simulink model "Viento_coordenadas"  (R2020a)
settings: Solver=VariableStepAuto  StartTime=0.0  StopTime=20  RelTol=1e-3
values from neighbouring files (symbols this model uses):
  Areavector = [0.293;0.022;0.022]    [Iteradorcompleto.m]    (also in Parametros_iniciales.m)
  body_rate_0 = [0;0;0]    [Iteradorcompleto.m]    (also in Parametros_iniciales.m)
  cd = 0.2    [Iteradorcompleto.m]    (also in Parametros_iniciales.m)
  Euler_0 = [0;0;0]    [Iteradorcompleto.m]    (also in Parametros_iniciales.m)
  g = [0;0;-3.66]    [Iteradorcompleto.m]    (also in Parametros_iniciales.m)
  I = [[0.01739,0,0];[0,0.01739,0];[0,0,0.0225]]    [Iteradorcompleto.m]    (also in Parametros_iniciales.m)
  m = T_V1toI*T_V2toV1*T_BtoV2    [Creacion_animacion.m]    (also in Iteradorcompleto.m = 2; Parametros_iniciales.m = 2)
  rho = 0.0195    [Iteradorcompleto.m]    (also in Parametros_iniciales.m)
  ts = 0.01    [Iteradorcompleto.m]    (also in Parametros_iniciales.m)
  vwind = real(-C*(log(1-probabilidad))^(1/K))    [DistribucionWeibul.m]    (also in Iteradorcompleto.m)
  XYZ_0 = [0;0;0]    [Iteradorcompleto.m]    (also in Parametros_iniciales.m = [0;0;5])
libraries: simulink x51, vrlib x2, aerolibutil x1
(part 4 of 4)

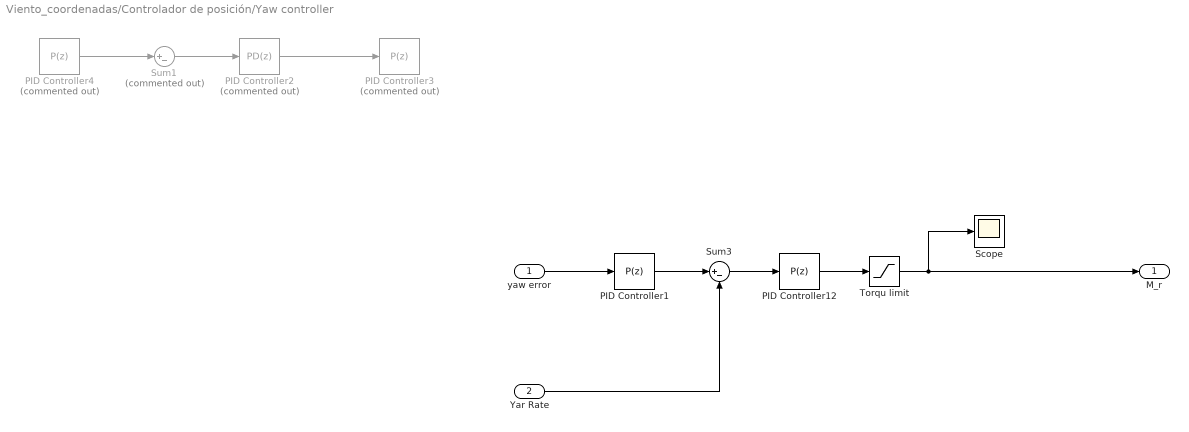
== system Viento_coordenadas/Controlador de posición/Yaw controller  ==
  yaw error : Inport
  Yar Rate : Inport  Port=2
  PID Controller1 : simulink/Continuous/PID Controller  Controller=P  Form=Parallel  TimeDomain=Discrete-time  UseExternalTs=off  SampleTime=ts  IntegratorMethod=Forward Euler  FilterMethod=Forward Euler  ControllerParametersSource=internal  P=4  I=1  D=0  UseFilter=on  N=100  TunerSelectOption=Transfer Function Based (PID Tuner App)  InitialConditionSource=internal  InitialConditionForIntegrator=0  InitialConditionForFilter=0  DifferentiatorICPrevScaledInput=0  ExternalReset=none  TrackingMode=off  Kt=1  LimitOutput=off  UpperSaturationLimit=inf  LowerSaturationLimit=-inf  LinearizeAsGain=on  AntiWindupMode=none  Kb=1  POutMin=[]  POutMax=[]  IOutMin=[]  IOutMax=[]  DOutMin=[]  DOutMax=[]  NOutMin=[]  NOutMax=[]  SumOutMin=[]  SumOutMax=[]  SaturationOutMin=[]  SaturationOutMax=[]  PParamMin=[]  PParamMax=[]  IParamMin=[]  IParamMax=[]  DParamMin=[]  DParamMax=[]  NParamMin=[]  NParamMax=[]  KbParamMin=[]  KbParamMax=[]  KtParamMin=[]  KtParamMax=[]  KbOutMin=[]  KbOutMax=[]  KtOutMin=[]  KtOutMax=[]  IntegratorOutMin=[]  IntegratorOutMax=[]  FilterOutMin=[]  FilterOutMax=[]  SumI1OutMin=[]  SumI1OutMax=[]  SumI2OutMin=[]  SumI2OutMax=[]  SumI3OutMin=[]  SumI3OutMax=[]  SumI4OutMin=[]  SumI4OutMax=[]  SumDOutMin=[]  SumDOutMax=[]  DifferentiatorOutMin=[]  DifferentiatorOutMax=[]  FilterDiffOutCoefMin=[]  FilterDiffOutCoefMax=[]  ReciprocalOutMin=[]  ReciprocalOutMax=[]  SumDenOutMin=[]  SumDenOutMax=[]  SumNumOutMin=[]  SumNumOutMax=[]  DivideOutMin=[]  DivideOutMax=[]  UdiffTsProdOutMin=[]  UdiffTsProdOutMax=[]  NTsProdOutMin=[]  NTsProdOutMax=[]  UintegralTsProdOutMin=[]  UintegralTsProdOutMax=[]  UngainTsProdOutMin=[]  UngainTsProdOutMax=[]  IntegratorContinuousStateAttributes=''  IntegratorStateMustResolveToSignalObject=off  IntegratorRTWStateStorageClass=Auto  FilterContinuousStateAttributes=''  FilterStateMustResolveToSignalObject=off  FilterRTWStateStorageClass=Auto  ParallelPVariant=InternalParameters  IdealPVariant=Disabled  IVariant=Disabled  DVariant=Disabled  IntegratorVariant=Disabled  SatVariant=Disabled  AWVariant=Disabled  PCopyVariant=Disabled  TRVariant=Disabled  FdbkBlocksVariant=Forward  IdealPFdbkVariant=Disabled  SatFdbkVariant=Disabled  DerivativeFilterVariant=Disabled  NVariant=Disabled  NCopyVariant=Disabled_SignalSpec  FilterICVariant=Disabled  IntegratorICVariant=Disabled  ExternalResetVariant=Disabled  TRSumVariant=Passthrough  SumFdbkVariant=Disabled  SumVariant=Passthrough_P  TsampFilterVariant=InternalTs  TsampNgainVariant=Passthrough  TsampIntegralVariant=Disabled_SignalSpec
  PID Controller12 : simulink/Continuous/PID Controller  Controller=P  Form=Parallel  TimeDomain=Discrete-time  UseExternalTs=off  SampleTime=ts  IntegratorMethod=Forward Euler  FilterMethod=Forward Euler  ControllerParametersSource=internal  P=1.5  I=0.0156974923564251  D=-0.0168622468908016  UseFilter=on  N=1.70578345077793  TunerSelectOption=Transfer Function Based (PID Tuner App)  InitialConditionSource=internal  InitialConditionForIntegrator=0  InitialConditionForFilter=0  DifferentiatorICPrevScaledInput=0  ExternalReset=none  TrackingMode=off  Kt=1  LimitOutput=off  UpperSaturationLimit=inf  LowerSaturationLimit=-inf  LinearizeAsGain=on  AntiWindupMode=none  Kb=1  POutMin=[]  POutMax=[]  IOutMin=[]  IOutMax=[]  DOutMin=[]  DOutMax=[]  NOutMin=[]  NOutMax=[]  SumOutMin=[]  SumOutMax=[]  SaturationOutMin=[]  SaturationOutMax=[]  PParamMin=[]  PParamMax=[]  IParamMin=[]  IParamMax=[]  DParamMin=[]  DParamMax=[]  NParamMin=[]  NParamMax=[]  KbParamMin=[]  KbParamMax=[]  KtParamMin=[]  KtParamMax=[]  KbOutMin=[]  KbOutMax=[]  KtOutMin=[]  KtOutMax=[]  IntegratorOutMin=[]  IntegratorOutMax=[]  FilterOutMin=[]  FilterOutMax=[]  SumI1OutMin=[]  SumI1OutMax=[]  SumI2OutMin=[]  SumI2OutMax=[]  SumI3OutMin=[]  SumI3OutMax=[]  SumI4OutMin=[]  SumI4OutMax=[]  SumDOutMin=[]  SumDOutMax=[]  DifferentiatorOutMin=[]  DifferentiatorOutMax=[]  FilterDiffOutCoefMin=[]  FilterDiffOutCoefMax=[]  ReciprocalOutMin=[]  ReciprocalOutMax=[]  SumDenOutMin=[]  SumDenOutMax=[]  SumNumOutMin=[]  SumNumOutMax=[]  DivideOutMin=[]  DivideOutMax=[]  UdiffTsProdOutMin=[]  UdiffTsProdOutMax=[]  NTsProdOutMin=[]  NTsProdOutMax=[]  UintegralTsProdOutMin=[]  UintegralTsProdOutMax=[]  UngainTsProdOutMin=[]  UngainTsProdOutMax=[]  IntegratorContinuousStateAttributes=''  IntegratorStateMustResolveToSignalObject=off  IntegratorRTWStateStorageClass=Auto  FilterContinuousStateAttributes=''  FilterStateMustResolveToSignalObject=off  FilterRTWStateStorageClass=Auto  ParallelPVariant=InternalParameters  IdealPVariant=Disabled  IVariant=Disabled  DVariant=Disabled  IntegratorVariant=Disabled  SatVariant=Disabled  AWVariant=Disabled  PCopyVariant=Disabled  TRVariant=Disabled  FdbkBlocksVariant=Forward  IdealPFdbkVariant=Disabled  SatFdbkVariant=Disabled  DerivativeFilterVariant=Disabled  NVariant=Disabled  NCopyVariant=Disabled_SignalSpec  FilterICVariant=Disabled  IntegratorICVariant=Disabled  ExternalResetVariant=Disabled  TRSumVariant=Passthrough  SumFdbkVariant=Disabled  SumVariant=Passthrough_P  TsampFilterVariant=InternalTs  TsampNgainVariant=Passthrough  TsampIntegralVariant=Disabled_SignalSpec
  PID Controller2 : simulink/Continuous/PID Controller  Commented=on  Controller=PD  Form=Parallel  TimeDomain=Discrete-time  UseExternalTs=off  SampleTime=ts  IntegratorMethod=Forward Euler  FilterMethod=Forward Euler  ControllerParametersSource=internal  P=06  I=1  D=0.4  UseFilter=on  N=10  TunerSelectOption=Transfer Function Based (PID Tuner App)  InitialConditionSource=internal  InitialConditionForIntegrator=0  InitialConditionForFilter=0  DifferentiatorICPrevScaledInput=0  ExternalReset=none  TrackingMode=off  Kt=1  LimitOutput=off  UpperSaturationLimit=inf  LowerSaturationLimit=-inf  LinearizeAsGain=on  AntiWindupMode=none  Kb=1  POutMin=[]  POutMax=[]  IOutMin=[]  IOutMax=[]  DOutMin=[]  DOutMax=[]  NOutMin=[]  NOutMax=[]  SumOutMin=[]  SumOutMax=[]  SaturationOutMin=[]  SaturationOutMax=[]  PParamMin=[]  PParamMax=[]  IParamMin=[]  IParamMax=[]  DParamMin=[]  DParamMax=[]  NParamMin=[]  NParamMax=[]  KbParamMin=[]  KbParamMax=[]  KtParamMin=[]  KtParamMax=[]  KbOutMin=[]  KbOutMax=[]  KtOutMin=[]  KtOutMax=[]  IntegratorOutMin=[]  IntegratorOutMax=[]  FilterOutMin=[]  FilterOutMax=[]  SumI1OutMin=[]  SumI1OutMax=[]  SumI2OutMin=[]  SumI2OutMax=[]  SumI3OutMin=[]  SumI3OutMax=[]  SumI4OutMin=[]  SumI4OutMax=[]  SumDOutMin=[]  SumDOutMax=[]  DifferentiatorOutMin=[]  DifferentiatorOutMax=[]  FilterDiffOutCoefMin=[]  FilterDiffOutCoefMax=[]  ReciprocalOutMin=[]  ReciprocalOutMax=[]  SumDenOutMin=[]  SumDenOutMax=[]  SumNumOutMin=[]  SumNumOutMax=[]  DivideOutMin=[]  DivideOutMax=[]  UdiffTsProdOutMin=[]  UdiffTsProdOutMax=[]  NTsProdOutMin=[]  NTsProdOutMax=[]  UintegralTsProdOutMin=[]  UintegralTsProdOutMax=[]  UngainTsProdOutMin=[]  UngainTsProdOutMax=[]  IntegratorContinuousStateAttributes=''  IntegratorStateMustResolveToSignalObject=off  IntegratorRTWStateStorageClass=Auto  FilterContinuousStateAttributes=''  FilterStateMustResolveToSignalObject=off  FilterRTWStateStorageClass=Auto  ParallelPVariant=InternalParameters  IdealPVariant=Disabled  IVariant=Disabled  DVariant=InternalParameters  IntegratorVariant=Disabled  SatVariant=Disabled  AWVariant=Disabled  PCopyVariant=Disabled  TRVariant=Disabled  FdbkBlocksVariant=Forward  IdealPFdbkVariant=Disabled  SatFdbkVariant=Disabled  DerivativeFilterVariant=ForwardEulerFilter  NVariant=InternalParameters  NCopyVariant=Disabled  FilterICVariant=InternalICsFilter  IntegratorICVariant=Disabled  ExternalResetVariant=Disabled  TRSumVariant=Passthrough  SumFdbkVariant=Disabled  SumVariant=Sum_PD  TsampFilterVariant=InternalTs  TsampNgainVariant=Passthrough  TsampIntegralVariant=Disabled_SignalSpec
  PID Controller3 : simulink/Continuous/PID Controller  Commented=on  Controller=P  Form=Parallel  TimeDomain=Discrete-time  UseExternalTs=off  SampleTime=ts  IntegratorMethod=Forward Euler  FilterMethod=Forward Euler  ControllerParametersSource=internal  P=0.7  I=1  D=0  UseFilter=on  N=100  TunerSelectOption=Transfer Function Based (PID Tuner App)  InitialConditionSource=internal  InitialConditionForIntegrator=0  InitialConditionForFilter=0  DifferentiatorICPrevScaledInput=0  ExternalReset=none  TrackingMode=off  Kt=1  LimitOutput=off  UpperSaturationLimit=inf  LowerSaturationLimit=-inf  LinearizeAsGain=on  AntiWindupMode=none  Kb=1  POutMin=[]  POutMax=[]  IOutMin=[]  IOutMax=[]  DOutMin=[]  DOutMax=[]  NOutMin=[]  NOutMax=[]  SumOutMin=[]  SumOutMax=[]  SaturationOutMin=[]  SaturationOutMax=[]  PParamMin=[]  PParamMax=[]  IParamMin=[]  IParamMax=[]  DParamMin=[]  DParamMax=[]  NParamMin=[]  NParamMax=[]  KbParamMin=[]  KbParamMax=[]  KtParamMin=[]  KtParamMax=[]  KbOutMin=[]  KbOutMax=[]  KtOutMin=[]  KtOutMax=[]  IntegratorOutMin=[]  IntegratorOutMax=[]  FilterOutMin=[]  FilterOutMax=[]  SumI1OutMin=[]  SumI1OutMax=[]  SumI2OutMin=[]  SumI2OutMax=[]  SumI3OutMin=[]  SumI3OutMax=[]  SumI4OutMin=[]  SumI4OutMax=[]  SumDOutMin=[]  SumDOutMax=[]  DifferentiatorOutMin=[]  DifferentiatorOutMax=[]  FilterDiffOutCoefMin=[]  FilterDiffOutCoefMax=[]  ReciprocalOutMin=[]  ReciprocalOutMax=[]  SumDenOutMin=[]  SumDenOutMax=[]  SumNumOutMin=[]  SumNumOutMax=[]  DivideOutMin=[]  DivideOutMax=[]  UdiffTsProdOutMin=[]  UdiffTsProdOutMax=[]  NTsProdOutMin=[]  NTsProdOutMax=[]  UintegralTsProdOutMin=[]  UintegralTsProdOutMax=[]  UngainTsProdOutMin=[]  UngainTsProdOutMax=[]  IntegratorContinuousStateAttributes=''  IntegratorStateMustResolveToSignalObject=off  IntegratorRTWStateStorageClass=Auto  FilterContinuousStateAttributes=''  FilterStateMustResolveToSignalObject=off  FilterRTWStateStorageClass=Auto  ParallelPVariant=InternalParameters  IdealPVariant=Disabled  IVariant=Disabled  DVariant=Disabled  IntegratorVariant=Disabled  SatVariant=Disabled  AWVariant=Disabled  PCopyVariant=Disabled  TRVariant=Disabled  FdbkBlocksVariant=Forward  IdealPFdbkVariant=Disabled  SatFdbkVariant=Disabled  DerivativeFilterVariant=Disabled  NVariant=Disabled  NCopyVariant=Disabled_SignalSpec  FilterICVariant=Disabled  IntegratorICVariant=Disabled  ExternalResetVariant=Disabled  TRSumVariant=Passthrough  SumFdbkVariant=Disabled  SumVariant=Passthrough_P  TsampFilterVariant=InternalTs  TsampNgainVariant=Passthrough  TsampIntegralVariant=Disabled_SignalSpec
  PID Controller4 : simulink/Continuous/PID Controller  Commented=on  Controller=P  Form=Parallel  TimeDomain=Discrete-time  UseExternalTs=off  SampleTime=ts  IntegratorMethod=Forward Euler  FilterMethod=Forward Euler  ControllerParametersSource=internal  P=6  I=1  D=0  UseFilter=on  N=100  TunerSelectOption=Transfer Function Based (PID Tuner App)  InitialConditionSource=internal  InitialConditionForIntegrator=0  InitialConditionForFilter=0  DifferentiatorICPrevScaledInput=0  ExternalReset=none  TrackingMode=off  Kt=1  LimitOutput=off  UpperSaturationLimit=inf  LowerSaturationLimit=-inf  LinearizeAsGain=on  AntiWindupMode=none  Kb=1  POutMin=[]  POutMax=[]  IOutMin=[]  IOutMax=[]  DOutMin=[]  DOutMax=[]  NOutMin=[]  NOutMax=[]  SumOutMin=[]  SumOutMax=[]  SaturationOutMin=[]  SaturationOutMax=[]  PParamMin=[]  PParamMax=[]  IParamMin=[]  IParamMax=[]  DParamMin=[]  DParamMax=[]  NParamMin=[]  NParamMax=[]  KbParamMin=[]  KbParamMax=[]  KtParamMin=[]  KtParamMax=[]  KbOutMin=[]  KbOutMax=[]  KtOutMin=[]  KtOutMax=[]  IntegratorOutMin=[]  IntegratorOutMax=[]  FilterOutMin=[]  FilterOutMax=[]  SumI1OutMin=[]  SumI1OutMax=[]  SumI2OutMin=[]  SumI2OutMax=[]  SumI3OutMin=[]  SumI3OutMax=[]  SumI4OutMin=[]  SumI4OutMax=[]  SumDOutMin=[]  SumDOutMax=[]  DifferentiatorOutMin=[]  DifferentiatorOutMax=[]  FilterDiffOutCoefMin=[]  FilterDiffOutCoefMax=[]  ReciprocalOutMin=[]  ReciprocalOutMax=[]  SumDenOutMin=[]  SumDenOutMax=[]  SumNumOutMin=[]  SumNumOutMax=[]  DivideOutMin=[]  DivideOutMax=[]  UdiffTsProdOutMin=[]  UdiffTsProdOutMax=[]  NTsProdOutMin=[]  NTsProdOutMax=[]  UintegralTsProdOutMin=[]  UintegralTsProdOutMax=[]  UngainTsProdOutMin=[]  UngainTsProdOutMax=[]  IntegratorContinuousStateAttributes=''  IntegratorStateMustResolveToSignalObject=off  IntegratorRTWStateStorageClass=Auto  FilterContinuousStateAttributes=''  FilterStateMustResolveToSignalObject=off  FilterRTWStateStorageClass=Auto  ParallelPVariant=InternalParameters  IdealPVariant=Disabled  IVariant=Disabled  DVariant=Disabled  IntegratorVariant=Disabled  SatVariant=Disabled  AWVariant=Disabled  PCopyVariant=Disabled  TRVariant=Disabled  FdbkBlocksVariant=Forward  IdealPFdbkVariant=Disabled  SatFdbkVariant=Disabled  DerivativeFilterVariant=Disabled  NVariant=Disabled  NCopyVariant=Disabled_SignalSpec  FilterICVariant=Disabled  IntegratorICVariant=Disabled  ExternalResetVariant=Disabled  TRSumVariant=Passthrough  SumFdbkVariant=Disabled  SumVariant=Passthrough_P  TsampFilterVariant=InternalTs  TsampNgainVariant=Passthrough  TsampIntegralVariant=Disabled_SignalSpec
  Scope : Scope
  Sum1 : Sum  Commented=on  Inputs=|+-
  Sum3 : Sum  Inputs=|+-
  Torqu limit : Saturate  UpperLimit=1  LowerLimit=-1
  M_r : Outport
  wires:
  PID Controller12/1 -> Torqu limit/1
  Sum3/1 -> PID Controller12/1
  PID Controller1/1 -> Sum3/1
  Torqu limit/1 -> M_r/1, Scope/1
  PID Controller4/1 -> Sum1/1
  Sum1/1 -> PID Controller2/1
  PID Controller2/1 -> PID Controller3/1
  yaw error/1 -> PID Controller1/1
  Yar Rate/1 -> Sum3/2

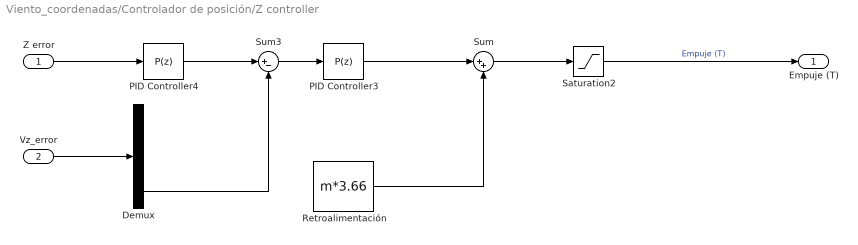
== system Viento_coordenadas/Controlador de posición/Z controller ==
  Z error : Inport
  Vz_error : Inport  Port=2
  Demux : Demux  Outputs=3
  PID Controller3 : simulink/Continuous/PID Controller  Controller=P  Form=Parallel  TimeDomain=Discrete-time  UseExternalTs=off  SampleTime=ts  IntegratorMethod=Forward Euler  FilterMethod=Forward Euler  ControllerParametersSource=internal  P=1.5  I=1  D=0  UseFilter=on  N=100  TunerSelectOption=Transfer Function Based (PID Tuner App)  InitialConditionSource=internal  InitialConditionForIntegrator=0  InitialConditionForFilter=0  DifferentiatorICPrevScaledInput=0  ExternalReset=none  TrackingMode=off  Kt=1  LimitOutput=off  UpperSaturationLimit=inf  LowerSaturationLimit=-inf  LinearizeAsGain=on  AntiWindupMode=none  Kb=1  POutMin=[]  POutMax=[]  IOutMin=[]  IOutMax=[]  DOutMin=[]  DOutMax=[]  NOutMin=[]  NOutMax=[]  SumOutMin=[]  SumOutMax=[]  SaturationOutMin=[]  SaturationOutMax=[]  PParamMin=[]  PParamMax=[]  IParamMin=[]  IParamMax=[]  DParamMin=[]  DParamMax=[]  NParamMin=[]  NParamMax=[]  KbParamMin=[]  KbParamMax=[]  KtParamMin=[]  KtParamMax=[]  KbOutMin=[]  KbOutMax=[]  KtOutMin=[]  KtOutMax=[]  IntegratorOutMin=[]  IntegratorOutMax=[]  FilterOutMin=[]  FilterOutMax=[]  SumI1OutMin=[]  SumI1OutMax=[]  SumI2OutMin=[]  SumI2OutMax=[]  SumI3OutMin=[]  SumI3OutMax=[]  SumI4OutMin=[]  SumI4OutMax=[]  SumDOutMin=[]  SumDOutMax=[]  DifferentiatorOutMin=[]  DifferentiatorOutMax=[]  FilterDiffOutCoefMin=[]  FilterDiffOutCoefMax=[]  ReciprocalOutMin=[]  ReciprocalOutMax=[]  SumDenOutMin=[]  SumDenOutMax=[]  SumNumOutMin=[]  SumNumOutMax=[]  DivideOutMin=[]  DivideOutMax=[]  UdiffTsProdOutMin=[]  UdiffTsProdOutMax=[]  NTsProdOutMin=[]  NTsProdOutMax=[]  UintegralTsProdOutMin=[]  UintegralTsProdOutMax=[]  UngainTsProdOutMin=[]  UngainTsProdOutMax=[]  IntegratorContinuousStateAttributes=''  IntegratorStateMustResolveToSignalObject=off  IntegratorRTWStateStorageClass=Auto  FilterContinuousStateAttributes=''  FilterStateMustResolveToSignalObject=off  FilterRTWStateStorageClass=Auto  ParallelPVariant=InternalParameters  IdealPVariant=Disabled  IVariant=Disabled  DVariant=Disabled  IntegratorVariant=Disabled  SatVariant=Disabled  AWVariant=Disabled  PCopyVariant=Disabled  TRVariant=Disabled  FdbkBlocksVariant=Forward  IdealPFdbkVariant=Disabled  SatFdbkVariant=Disabled  DerivativeFilterVariant=Disabled  NVariant=Disabled  NCopyVariant=Disabled_SignalSpec  FilterICVariant=Disabled  IntegratorICVariant=Disabled  ExternalResetVariant=Disabled  TRSumVariant=Passthrough  SumFdbkVariant=Disabled  SumVariant=Passthrough_P  TsampFilterVariant=InternalTs  TsampNgainVariant=Passthrough  TsampIntegralVariant=Disabled_SignalSpec
  PID Controller4 : simulink/Continuous/PID Controller  Controller=P  Form=Parallel  TimeDomain=Discrete-time  UseExternalTs=off  SampleTime=ts  IntegratorMethod=Forward Euler  FilterMethod=Forward Euler  ControllerParametersSource=internal  P=0.4  I=1  D=0  UseFilter=on  N=100  TunerSelectOption=Transfer Function Based (PID Tuner App)  InitialConditionSource=internal  InitialConditionForIntegrator=0  InitialConditionForFilter=0  DifferentiatorICPrevScaledInput=0  ExternalReset=none  TrackingMode=off  Kt=1  LimitOutput=off  UpperSaturationLimit=inf  LowerSaturationLimit=-inf  LinearizeAsGain=on  AntiWindupMode=none  Kb=1  POutMin=[]  POutMax=[]  IOutMin=[]  IOutMax=[]  DOutMin=[]  DOutMax=[]  NOutMin=[]  NOutMax=[]  SumOutMin=[]  SumOutMax=[]  SaturationOutMin=[]  SaturationOutMax=[]  PParamMin=[]  PParamMax=[]  IParamMin=[]  IParamMax=[]  DParamMin=[]  DParamMax=[]  NParamMin=[]  NParamMax=[]  KbParamMin=[]  KbParamMax=[]  KtParamMin=[]  KtParamMax=[]  KbOutMin=[]  KbOutMax=[]  KtOutMin=[]  KtOutMax=[]  IntegratorOutMin=[]  IntegratorOutMax=[]  FilterOutMin=[]  FilterOutMax=[]  SumI1OutMin=[]  SumI1OutMax=[]  SumI2OutMin=[]  SumI2OutMax=[]  SumI3OutMin=[]  SumI3OutMax=[]  SumI4OutMin=[]  SumI4OutMax=[]  SumDOutMin=[]  SumDOutMax=[]  DifferentiatorOutMin=[]  DifferentiatorOutMax=[]  FilterDiffOutCoefMin=[]  FilterDiffOutCoefMax=[]  ReciprocalOutMin=[]  ReciprocalOutMax=[]  SumDenOutMin=[]  SumDenOutMax=[]  SumNumOutMin=[]  SumNumOutMax=[]  DivideOutMin=[]  DivideOutMax=[]  UdiffTsProdOutMin=[]  UdiffTsProdOutMax=[]  NTsProdOutMin=[]  NTsProdOutMax=[]  UintegralTsProdOutMin=[]  UintegralTsProdOutMax=[]  UngainTsProdOutMin=[]  UngainTsProdOutMax=[]  IntegratorContinuousStateAttributes=''  IntegratorStateMustResolveToSignalObject=off  IntegratorRTWStateStorageClass=Auto  FilterContinuousStateAttributes=''  FilterStateMustResolveToSignalObject=off  FilterRTWStateStorageClass=Auto  ParallelPVariant=InternalParameters  IdealPVariant=Disabled  IVariant=Disabled  DVariant=Disabled  IntegratorVariant=Disabled  SatVariant=Disabled  AWVariant=Disabled  PCopyVariant=Disabled  TRVariant=Disabled  FdbkBlocksVariant=Forward  IdealPFdbkVariant=Disabled  SatFdbkVariant=Disabled  DerivativeFilterVariant=Disabled  NVariant=Disabled  NCopyVariant=Disabled_SignalSpec  FilterICVariant=Disabled  IntegratorICVariant=Disabled  ExternalResetVariant=Disabled  TRSumVariant=Passthrough  SumFdbkVariant=Disabled  SumVariant=Passthrough_P  TsampFilterVariant=InternalTs  TsampNgainVariant=Passthrough  TsampIntegralVariant=Disabled_SignalSpec
  "Retroalimentación " : Constant  Value=m*3.66
  Saturation2 : Saturate  UpperLimit=11.396  LowerLimit=-11.396
  Sum : Sum  Inputs=|++
  Sum3 : Sum  Inputs=|+-
  Empuje (T) : Outport
  wires:
  PID Controller4/1 -> Sum3/1
  Sum3/1 -> PID Controller3/1
  Demux/3 -> Sum3/2
  Saturation2/1 -> Empuje (T)/1  "Empuje (T)"
  Sum/1 -> Saturation2/1
  "Retroalimentación "/1 -> Sum/2
  Z error/1 -> PID Controller4/1
  Vz_error/1 -> Demux/1
  PID Controller3/1 -> Sum/1

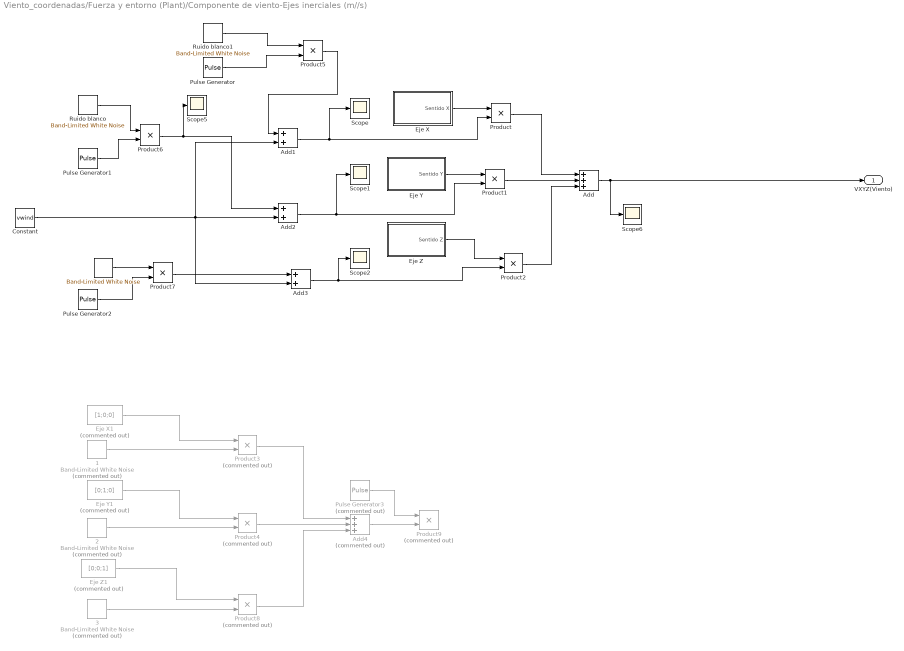
== system Viento_coordenadas/Fuerza y entorno (Plant)/Componente de viento-Ejes inerciales (m//s) ==
  " " : simulink/Sources/Band-Limited White Noise  Cov=[0.05]  Ts=10  seed=[13244]
  " 1" : simulink/Sources/Band-Limited White Noise  Commented=on  Cov=[0.05]  Ts=10  seed=[13244]
  " 2" : simulink/Sources/Band-Limited White Noise  Commented=on  Cov=[0.05]  Ts=10  seed=[13244]
  " 3" : simulink/Sources/Band-Limited White Noise  Commented=on  Cov=[0.05]  Ts=10  seed=[13244]
  Add : Sum  Inputs=+++
  Add1 : Sum
  Add2 : Sum
  Add3 : Sum
  Add4 : Sum  Commented=on  Inputs=+++
  Constant : Constant  Value=vwind
  Eje X : Subsystem
  Eje X1 : Constant  Commented=on  Value=[1;0;0]
  Eje Y : Subsystem
  Eje Y1 : Constant  Commented=on  Value=[0;1;0]
  Eje Z : Subsystem
  Eje Z1 : Constant  Commented=on  Value=[0;0;1]
  Product{,1..2,5..7} (6 alike) : Product
  Product{3..4,8..9} (4 alike) : Product  Commented=on
  Pulse Generator : DiscretePulseGenerator  PulseType=Time based  Amplitude=0.5  Period=5  PulseWidth=20
  Pulse Generator1 : DiscretePulseGenerator  PulseType=Time based  Period=5  PulseWidth=25
  Pulse Generator2 : DiscretePulseGenerator  PulseType=Time based  Amplitude=0.5  Period=5  PulseWidth=17
  Pulse Generator3 : DiscretePulseGenerator  Commented=on  PulseType=Time based  Period=5  PulseWidth=90
  Ruido blanco : simulink/Sources/Band-Limited White Noise  Cov=[0.05]  Ts=7  seed=[23341]
  Ruido blanco1 : simulink/Sources/Band-Limited White Noise  Cov=[0.05]  Ts=5  seed=[23341]
  Scope{,1..2,5..6} (5 alike) : Scope
  VXYZ(Viento) : Outport
  wires:
  Product/1 -> Add/1
  Constant/1 -> Add3/2, Add2/2, Add1/2
  Add1/1 -> Scope/1, Product/2
  Add2/1 -> Scope1/1, Product1/2
  Add3/1 -> Scope2/1, Product2/2
  Ruido blanco1/1 -> Product5/1
  Pulse Generator/1 -> Product5/2
  Product5/1 -> Add1/1
  Ruido blanco/1 -> Product6/1
  Product6/1 -> Scope5/1, Add2/1
  " "/1 -> Product7/1
  Product7/1 -> Add3/1
  Pulse Generator1/1 -> Product6/2
  Pulse Generator2/1 -> Product7/2
  " 1"/1 -> Product3/2
  Eje X1/1 -> Product3/1
  " 2"/1 -> Product4/2
  Eje Y1/1 -> Product4/1
  " 3"/1 -> Product8/2
  Eje Z1/1 -> Product8/1
  Product4/1 -> Add4/2
  Product3/1 -> Add4/1
  Product8/1 -> Add4/3
  Add4/1 -> Product9/2
  Pulse Generator3/1 -> Product9/1
  Add/1 -> Scope6/1, VXYZ(Viento)/1
  Eje X/1(Sentido X) -> Product/1
  Eje Y/1(Sentido Y) -> Product1/1
  Eje Z/1(Sentido Z) -> Product2/1
  Product1/1 -> Add/2
  Product2/1 -> Add/3

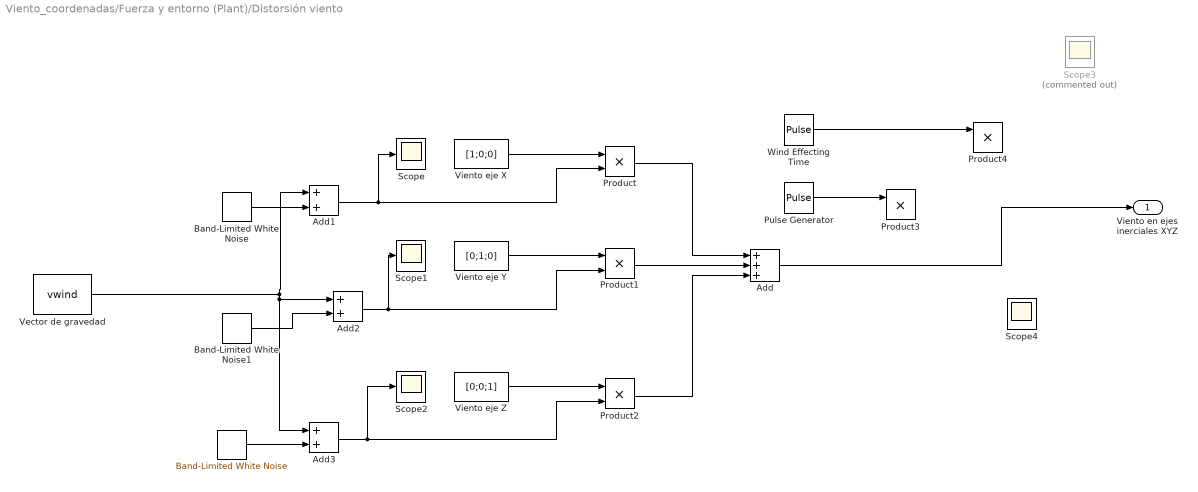
== system Viento_coordenadas/Fuerza y entorno (Plant)/Distorsión viento ==
  " " : simulink/Sources/Band-Limited White Noise  Cov=[0.5]  Ts=5  seed=[13244]
  Add : Sum  Inputs=+++
  Add1 : Sum
  Add2 : Sum
  Add3 : Sum
  Band-Limited White Noise : simulink/Sources/Band-Limited White Noise  Cov=[0.5]  Ts=5  seed=[23341]
  Band-Limited White Noise1 : simulink/Sources/Band-Limited White Noise  Cov=[0.5]  Ts=5  seed=[41323]
  Product{,1..4} (5 alike) : Product
  Pulse Generator : DiscretePulseGenerator  PulseType=Time based  Period=2.5  PulseWidth=40
  Scope{,1..2,4} (4 alike) : Scope
  Scope3 : Scope  Commented=on
  Vector de gravedad : Constant  Value=vwind  SampleTime=-1
  Viento eje X : Constant  Value=[1;0;0]
  Viento eje Y : Constant  Value=[0;1;0]
  Viento eje Z : Constant  Value=[0;0;1]
  Wind Effecting Time : DiscretePulseGenerator  PulseType=Time based  Period=100  PulseWidth=10
  Viento en ejes inerciales XYZ : Outport
  wires:
  Viento eje X/1 -> Product/1
  Viento eje Y/1 -> Product1/1
  Viento eje Z/1 -> Product2/1
  Product1/1 -> Add/2
  Product/1 -> Add/1
  Product2/1 -> Add/3
  Pulse Generator/1 -> Product3/1
  Wind Effecting Time/1 -> Product4/1
  Add/1 -> Viento en ejes inerciales XYZ/1
  Band-Limited White Noise/1 -> Add1/2
  Add1/1 -> Scope/1, Product/2
  Band-Limited White Noise1/1 -> Add2/2
  Add2/1 -> Scope1/1, Product1/2
  " "/1 -> Add3/2
  Add3/1 -> Scope2/1, Product2/2
  Vector de gravedad/1 -> Add3/1, Add2/1, Add1/1

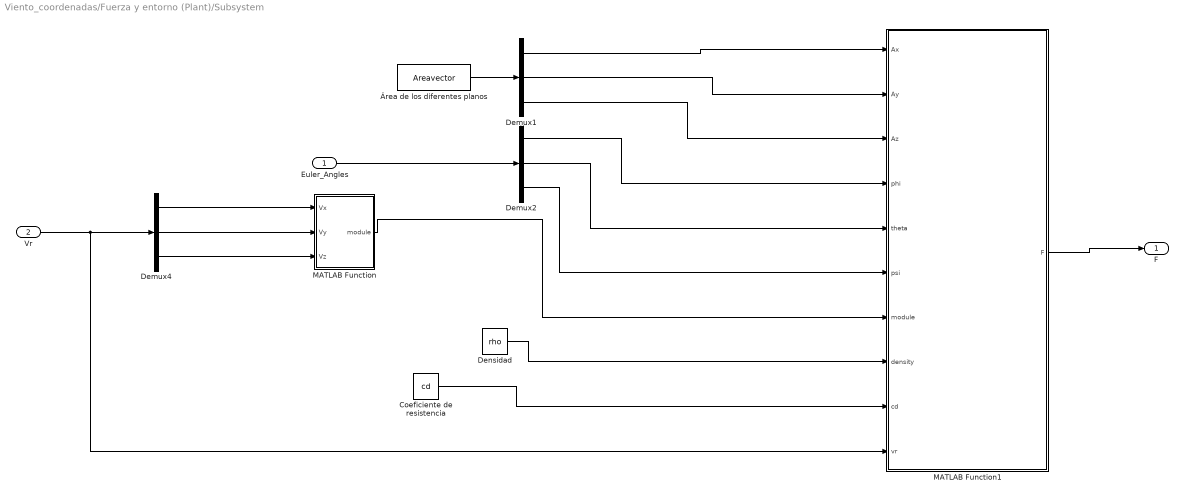
== system Viento_coordenadas/Fuerza y entorno (Plant)/Subsystem ==
  Euler_Angles : Inport
  Vr : Inport  Port=2
  Coeficiente de resistencia : Constant  Value=cd  SampleTime=-1
  Demux1 : Demux  Outputs=3
  Demux2 : Demux  Outputs=3
  Demux4 : Demux  Outputs=3
  Densidad : Constant  Value=rho  SampleTime=-1
  MATLAB Function : MATLAB Function  TreatAsAtomicUnit=on
  MATLAB Function1 : MATLAB Function  TreatAsAtomicUnit=on
  Área de los diferentes planos : Constant  Value=Areavector  SampleTime=-1
  F : Outport
  wires:
  Demux4/3 -> MATLAB Function/3(Vz)
  Demux4/2 -> MATLAB Function/2(Vy)
  Demux2/3 -> MATLAB Function1/6(psi)
  MATLAB Function1/1(F) -> F/1
  Área de los diferentes planos/1 -> Demux1/1
  Demux1/2 -> MATLAB Function1/2(Ay)
  Demux1/3 -> MATLAB Function1/3(Az)
  Euler_Angles/1 -> Demux2/1
  Demux1/1 -> MATLAB Function1/1(Ax)
  Demux2/1 -> MATLAB Function1/4(phi)
  Demux2/2 -> MATLAB Function1/5(theta)
  MATLAB Function/1(module) -> MATLAB Function1/7(module)
  Densidad/1 -> MATLAB Function1/8(density)
  Vr/1 -> Demux4/1, MATLAB Function1/10(vr)
  Demux4/1 -> MATLAB Function/1(Vx)
  Coeficiente de resistencia/1 -> MATLAB Function1/9(cd)

== system Viento_coordenadas/Fuerza y entorno (Plant)/Componente de viento-Ejes inerciales (m//s)/Eje X ==
  Eje X : Constant  Value=[-1;0;0]
  Eje X2 : Constant  Value=[-1;0;0]
  Product : Product
  Pulse Generator : DiscretePulseGenerator  PulseType=Time based  Amplitude=0.5  Period=10  PulseWidth=80
  Ruido blanco2 : simulink/Sources/Band-Limited White Noise  Cov=[0.05]  Ts=6  seed=[23341]
  Switch : Switch  Criteria=u2 > Threshold  Threshold=0.01
  Sentido X : Outport
  wires:
  Ruido blanco2/1 -> Product/1
  Pulse Generator/1 -> Product/2
  Switch/1 -> Sentido X/1
  Eje X/1 -> Switch/1
  Eje X2/1 -> Switch/3
  Product/1 -> Switch/2

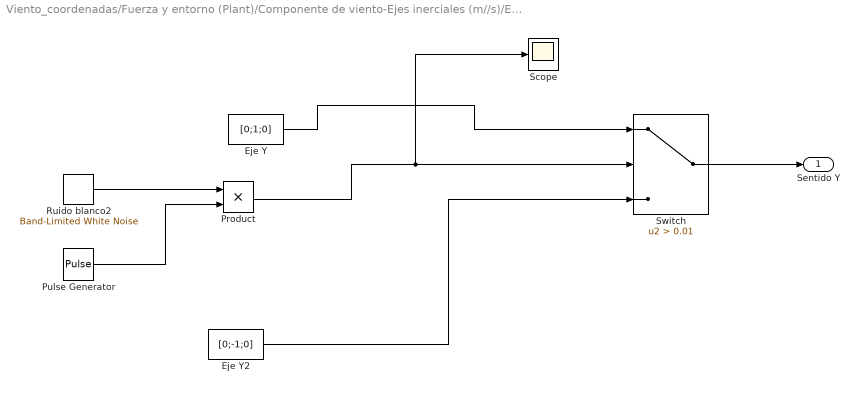
== system Viento_coordenadas/Fuerza y entorno (Plant)/Componente de viento-Ejes inerciales (m//s)/Eje Y ==
  Eje Y : Constant  Value=[0;1;0]
  Eje Y2 : Constant  Value=[0;-1;0]
  Product : Product
  Pulse Generator : DiscretePulseGenerator  PulseType=Time based  Amplitude=0.5  Period=10  PulseWidth=80
  Ruido blanco2 : simulink/Sources/Band-Limited White Noise  Cov=[0.05]  Ts=7  seed=[23341]
  Scope : Scope
  Switch : Switch  Criteria=u2 > Threshold  Threshold=0.01
  Sentido Y : Outport
  wires:
  Eje Y2/1 -> Switch/3
  Eje Y/1 -> Switch/1
  Switch/1 -> Sentido Y/1
  Ruido blanco2/1 -> Product/1
  Product/1 -> Scope/1, Switch/2
  Pulse Generator/1 -> Product/2

== system Viento_coordenadas/Fuerza y entorno (Plant)/Componente de viento-Ejes inerciales (m//s)/Eje Z ==
  Eje Z : Constant  Value=[0;0;1]
  Eje Z2 : Constant  Value=[0;0;-1]
  Product : Product
  Pulse Generator : DiscretePulseGenerator  PulseType=Time based  Amplitude=0.5  Period=10  PulseWidth=80
  Ruido blanco2 : simulink/Sources/Band-Limited White Noise  Cov=[0.05]  Ts=8  seed=[23341]
  Switch : Switch  Criteria=u2 > Threshold  Threshold=0.01
  Sentido Z : Outport
  wires:
  Eje Z2/1 -> Switch/3
  Eje Z/1 -> Switch/1
  Switch/1 -> Sentido Z/1
  Ruido blanco2/1 -> Product/1
  Product/1 -> Switch/2
  Pulse Generator/1 -> Product/2

== matlab function Viento_coordenadas/Controlador de Actitud/BtoITransform ==
  data: phi input; m output; theta input; psi input
function m = fcn(phi,theta,psi)
    T_BtoV2 = [[1 0 0];[0 cos(-phi) sin(-phi)];[0 -sin(-phi) cos(-phi)]];
    T_V2toV1 = [[cos(-theta) 0 -sin(-theta)];[0 1 0];[sin(-theta) 0 cos(-theta)]];
    T_V1toI = [[cos(-psi) sin(-psi) 0];[-sin(-psi) cos(-psi) 0];[0 0 1]];
    m = T_V1toI*T_V2toV1*T_BtoV2;

== matlab function Viento_coordenadas/Controlador de Actitud/euler_rate ==
  data: p input; phi_d output; q input; r input; phi input; theta input; theta_d output; psi_d output; psi input
function [phi_d,theta_d,psi_d] = fcn(p,q,r,phi,theta,psi)
    D = [[1 sin(phi)*tan(theta) cos(phi)*tan(theta)];
         [0 cos(phi) -sin(phi)];
         [0 sin(phi)/cos(theta) cos(phi)/cos(theta)]];
    euler_rate = D*[p;q;r]
    phi_d = euler_rate(1)
    theta_d = euler_rate(2)
    psi_d = euler_rate(3)

== matlab function Viento_coordenadas/Controlador de posición/MATLAB Function ==
  data: Xe input; xb output; Ye input; psi input; yb output
function [xb,yb] = fcn(Xe,Ye,psi)
    m = [[cos(psi) sin(psi)];[-sin(psi) cos(psi)]]
    pos = m*[Xe;Ye]
    xb = pos(1)
    yb = pos(2)

== matlab function Viento_coordenadas/XYZsignal ==
  data: Xcmd input; RefXYZ output; Ycmd input; Zcmd input
function RefXYZ = fcn(Xcmd,Ycmd,Zcmd)

RefXYZ = [Xcmd;Ycmd;Zcmd]

== matlab function Viento_coordenadas/Controlador de Actitud/ItoBTransform ==
  data: phi input; m output; theta input; psi input
function m = fcn(phi,theta,psi)
    T_ItoV1 = [[cos(psi) sin(psi) 0];[-sin(psi) cos(psi) 0];[0 0 1]]; 
    T_V1toV2 = [[cos(theta) 0 -sin(theta)];[0 1 0];[sin(theta) 0 cos(theta)]];
    T_V2toB = [[1 0 0];[0 cos(phi) sin(phi)];[0 -sin(phi) cos(phi)]];
    m = T_V2toB*T_V1toV2*T_ItoV1

== matlab function Viento_coordenadas/Rumbo ==
  data: VXYZ1 input; VXYZ2 input; y output; psi input
function y = fcn(VXYZ1,VXYZ2,psi)
    veloc = [VXYZ1;VXYZ2];
    matrix = [cos(psi) sin(psi);-sin(psi) cos(psi)];
    vbody = matrix*veloc;
      
    y = atan2(vbody(2),vbody(1));

== matlab function Viento_coordenadas/Fuerza y entorno (Plant)/Subsystem/MATLAB Function ==
  data: Vx input; module output; Vy input; Vz input
function module = fcn(Vx,Vy,Vz)

module = sqrt(Vx^(2)+Vy^(2)+Vz^(2));

== matlab function Viento_coordenadas/Modo de vuelo ==
  data: clock input; mode output
function mode = fcn(clock)
if clock < 1
    mode = 0
else
    mode = 1    
end

== matlab function Viento_coordenadas/Fuerza y entorno (Plant)/Subsystem/MATLAB Function1 ==
  data: Ax input; F output; Ay input; Az input; phi input; theta input; psi input; module input; density input; cd input; vr input
function F = fcn(Ax,Ay,Az,phi,theta,psi,module,density,cd,vr)
    Ixb = [cos(theta)*cos(psi) ; cos(theta)*sin(psi) ; -sin(theta)]';
    Iyb = [sin(phi)*sin(theta)*cos(psi)-cos(phi)*sin(psi); sin(phi)*sin(theta)*sin(psi)+cos(phi)*cos(psi) ; sin(phi)*cos(theta)]';
    Izb = [cos(phi)*sin(theta)*cos(psi)+sin(phi)*sin(psi); cos(phi)*sin(theta)*sin(psi)-sin(phi)*cos(psi) ; cos(phi)*cos(theta)]';
    
    A1 = Ax*abs(Ixb*vr/module);
    A2 = Ay*abs(Iyb*vr/module);
    A3 = Az*abs(Izb*vr/module);
    A = A1+A2+A3;

F = 0.5*cd*density*module*A*vr
